simulink model "DPendulum_Simulink"  (R2023a)
settings: Solver=VariableStepAuto  StartTime=0.0  StopTime=5  RelTol=1e-3
settings Model: Creator=Inovicht  LastModifiedBy=Inovicht

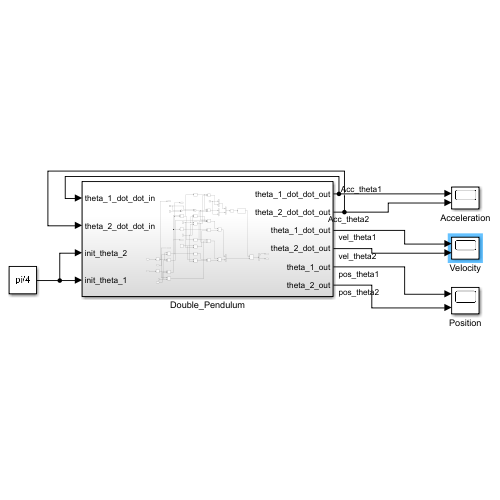
[thumbnail: Simulink's stored preview of the top-level diagram]
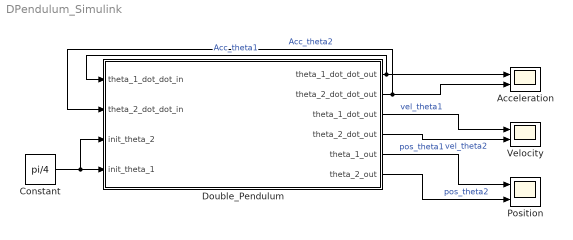
== system DPendulum_Simulink ==
  Acceleration : Scope  NumInputPorts=2
  Constant : Constant  Value=pi/4
  Double_Pendulum : Subsystem
  Position : Scope  NumInputPorts=2
  Velocity : Scope  NumInputPorts=2
  wires:
  Constant/1 -> Double_Pendulum/3(init_theta_2), Double_Pendulum/4(init_theta_1)
  Double_Pendulum/1(theta_1_dot_dot_out) -> Double_Pendulum/1(theta_1_dot_dot_in), Acceleration/1  "Acc_theta1"
  Double_Pendulum/3(theta_1_dot_out) -> Velocity/1  "vel_theta1"
  Double_Pendulum/2(theta_2_dot_dot_out) -> Acceleration/2, Double_Pendulum/2(theta_2_dot_dot_in)  "Acc_theta2"
  Double_Pendulum/6(theta_2_out) -> Position/2  "pos_theta2"
  Double_Pendulum/5(theta_1_out) -> Position/1  "pos_theta1"
  Double_Pendulum/4(theta_2_dot_out) -> Velocity/2  "vel_theta2"

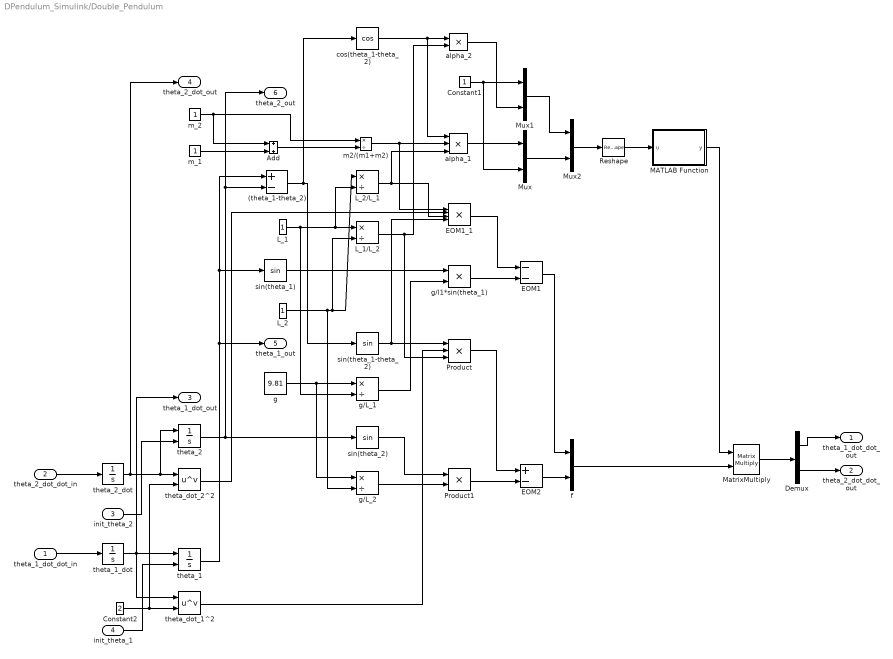
== system DPendulum_Simulink/Double_Pendulum ==
  theta_1_dot_dot_in : Inport
  theta_2_dot_dot_in : Inport  Port=2
  init_theta_2 : Inport  Port=3
  init_theta_1 : Inport  Port=4
  (theta_1-theta_2) : Sum  Inputs=+-
  Add : Sum
  Constant1 : Constant
  Constant2 : Constant  Value=2
  Demux : Demux  Outputs=2
  EOM1 : Sum  Inputs=--
  EOM1_1 : Product  Inputs=4
  EOM2 : Sum  Inputs=+-
  L_1 : Constant
  L_1/L_2 : Product  Inputs=*/
  L_2 : Constant
  L_2/L_1 : Product  Inputs=*/
  MATLAB Function : MATLAB Function  TreatAsAtomicUnit=on
  MatrixMultiply : Product  Multiplication=Matrix(*)
  Mux : Mux  Inputs=2
  Mux1 : Mux  Inputs=2
  Mux2 : Mux  Inputs=2
  Product : Product  Inputs=3
  Product1 : Product
  Reshape : Reshape  OutputDimensionality=Customize  OutputDimensions=[2,2]
  alpha_1 : Product  Inputs=3
  alpha_2 : Product
  cos(theta_1-theta_2) : Trigonometry  Operator=cos
  f : Mux  Inputs=2
  g : Constant  Value=9.81
  g/L_1 : Product  Inputs=*/
  g/L_2 : Product  Inputs=*/
  g/l1*sin(theta_1) : Product
  m2/(m1+m2) : Product  Inputs=*/
  m_1 : Constant
  m_2 : Constant
  sin(theta_1) : Trigonometry
  sin(theta_1-theta_2) : Trigonometry
  sin(theta_2) : Trigonometry
  theta_1 : Integrator  InitialConditionSource=external  InitialCondition=pi/4
  theta_1_dot : Integrator
  theta_2 : Integrator  InitialConditionSource=external  InitialCondition=pi/4
  theta_2_dot : Integrator
  theta_dot_1^2 : Math  Operator=pow
  theta_dot_2^2 : Math  Operator=pow
  theta_1_dot_dot_out : Outport
  theta_2_dot_dot_out : Outport  Port=2
  theta_1_dot_out : Outport  Port=3
  theta_2_dot_out : Outport  Port=4
  theta_1_out : Outport  Port=5
  theta_2_out : Outport  Port=6
  wires:
  theta_1_dot_dot_in/1 -> theta_1_dot/1
  Product1/1 -> EOM2/2
  theta_2_dot_dot_in/1 -> theta_2_dot/1
  Product/1 -> EOM2/1
  theta_2_dot/1 -> theta_dot_2^2/1, theta_2/1, theta_2_dot_out/1
  init_theta_1/1 -> theta_1/2
  alpha_1/1 -> Mux/1
  init_theta_2/1 -> theta_2/2
  L_1/L_2/1 -> alpha_2/2, Product/3
  theta_1/1 -> (theta_1-theta_2)/1, sin(theta_1)/1, theta_1_out/1
  theta_1_dot/1 -> theta_dot_1^2/1, theta_1/1, theta_1_dot_out/1
  Constant2/1 -> theta_dot_1^2/2, theta_dot_2^2/2
  m_2/1 -> m2/(m1+m2)/1, Add/1
  m_1/1 -> Add/2
  Constant1/1 -> Mux/2, Mux1/1
  alpha_2/1 -> Mux1/2
  theta_2/1 -> (theta_1-theta_2)/2, theta_2_out/1, sin(theta_2)/1
  theta_dot_2^2/1 -> EOM1_1/2
  theta_dot_1^2/1 -> Product/2
  EOM1/1 -> f/1
  Add/1 -> m2/(m1+m2)/2
  L_2/1 -> L_1/L_2/2, L_2/L_1/1, g/L_2/2
  (theta_1-theta_2)/1 -> sin(theta_1-theta_2)/1, cos(theta_1-theta_2)/1
  MATLAB Function/1(y) -> MatrixMultiply/1
  L_1/1 -> L_2/L_1/2, L_1/L_2/1, g/L_1/2
  sin(theta_1)/1 -> g/l1*sin(theta_1)/1
  g/1 -> g/L_2/1, g/L_1/1
  m2/(m1+m2)/1 -> alpha_1/2, EOM1_1/1
  cos(theta_1-theta_2)/1 -> alpha_1/1, alpha_2/1
  EOM2/1 -> f/2
  L_2/L_1/1 -> EOM1_1/3, alpha_1/3
  sin(theta_1-theta_2)/1 -> EOM1_1/4, Product/1
  Mux/1 -> Mux2/2
  g/L_1/1 -> g/l1*sin(theta_1)/2
  g/l1*sin(theta_1)/1 -> EOM1/2
  sin(theta_2)/1 -> Product1/1
  g/L_2/1 -> Product1/2
  Demux/1 -> theta_1_dot_dot_out/1
  EOM1_1/1 -> EOM1/1
  Mux1/1 -> Mux2/1
  Mux2/1 -> Reshape/1
  f/1 -> MatrixMultiply/2
  Reshape/1 -> MATLAB Function/1(u)
  MatrixMultiply/1 -> Demux/1
  Demux/2 -> theta_2_dot_dot_out/1

== matlab function DPendulum_Simulink/Double_Pendulum/MATLAB Function ==
  data: u input; y output
function y = inverse_2x2(u)
    % u is a 2x2 matrix
    y = inv(u);
end
